simulink model "VSG_2M"  (R2022b)
settings: Solver=FixedStepAuto  StartTime=0.0  StopTime=2  FixedStep=1e-6  RelTol=1e-3
model workspace (MAT data in the model file):
  C = 0.0003
  D = 500
  GP = 0.6
  GQ = 20
  J = 2
  KQ = 0.06
  Kf = 80000
  Kv = 577
  L = 0.001
  Pref = 2000000
  Qref = 0
  Ts = 0.0001
  Ts_Power = 1e-06
  Ug = 400
  Vdc = 1000
  fsw = 20000
  t0 = 0.5
  tco = 1.3
  tf = 1.2
  wn = 314.159265359
undefined symbols (not defined in the file): DiscIntNeverNeededParam, Ion, Lithium
libraries: spsSeriesRLCBranchLib x8, spsFirstOrderFilterLib x7, spsMeanLib x5, slpidlib x5, spsabctodq0Lib x4, spsStairGeneratorLib x4, spsDiodeLib x4, spsPWMGeneratorDCDCLib x3, spsThreePhaseVIMeasurementLib x3, spsThreePhaseSeriesRLCBranchLib x3, spsPowerPositiveSequenceLib x2, spsBoostConverterLib x2
(part 2 of 2)

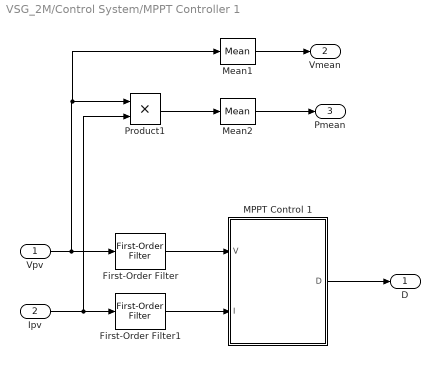
== system VSG_2M/Control System/MPPT Controller 1 ==
  Vpv : Inport
  Ipv : Inport  Port=2
  First-Order Filter : spsFirstOrderFilterLib/First-Order Filter  FilterType=Lowpass  Tc=1/Fc  Ts=Ts  Initialize=off  Vac_Init=[0, 0, 60]  Vdc_Init=0  PlotResponse=off  FreqRange="[0,  200,  1]"
  First-Order Filter1 : spsFirstOrderFilterLib/First-Order Filter  FilterType=Lowpass  Tc=1/Fc  Ts=Ts  Initialize=off  Vac_Init=[0, 0, 60]  Vdc_Init=0  PlotResponse=off  FreqRange="[0,  200,  1]"
  "MPPT Control 1 " : MATLAB Function  TreatAsAtomicUnit=on
  Mean1 : spsMeanLib/Mean  Freq=60  Vinit=650  Ts=Ts
  Mean2 : spsMeanLib/Mean  Freq=60  Vinit=1500e3  Ts=Ts
  Product1 : Product
  D : Outport  VectorParamsAs1DForOutWhenUnconnected=off
  Vmean : Outport  Port=2  VectorParamsAs1DForOutWhenUnconnected=off
  Pmean : Outport  Port=3  VectorParamsAs1DForOutWhenUnconnected=off
  wires:
  First-Order Filter1/1 -> "MPPT Control 1 "/2(I)
  First-Order Filter/1 -> "MPPT Control 1 "/1(V)
  Ipv/1 -> Product1/2, First-Order Filter1/1
  Vpv/1 -> Mean1/1, Product1/1, First-Order Filter/1
  "MPPT Control 1 "/1(D) -> D/1
  Product1/1 -> Mean2/1
  Mean1/1 -> Vmean/1
  Mean2/1 -> Pmean/1

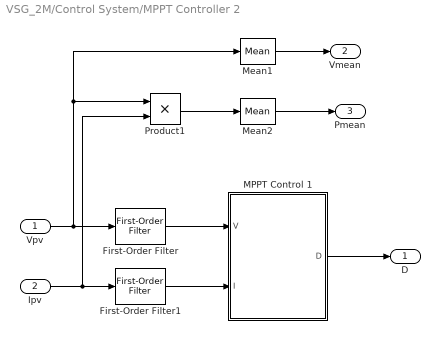
== system VSG_2M/Control System/MPPT Controller 2 ==
  Vpv : Inport
  Ipv : Inport  Port=2
  First-Order Filter : spsFirstOrderFilterLib/First-Order Filter  FilterType=Lowpass  Tc=1/Fc  Ts=Ts  Initialize=off  Vac_Init=[0, 0, 60]  Vdc_Init=0  PlotResponse=off  FreqRange="[0,  200,  1]"
  First-Order Filter1 : spsFirstOrderFilterLib/First-Order Filter  FilterType=Lowpass  Tc=1/Fc  Ts=Ts  Initialize=off  Vac_Init=[0, 0, 60]  Vdc_Init=0  PlotResponse=off  FreqRange="[0,  200,  1]"
  "MPPT Control 1 " : MATLAB Function  TreatAsAtomicUnit=on
  Mean1 : spsMeanLib/Mean  Freq=60  Vinit=420  Ts=Ts
  Mean2 : spsMeanLib/Mean  Freq=60  Vinit=500e3  Ts=Ts
  Product1 : Product
  D : Outport  VectorParamsAs1DForOutWhenUnconnected=off
  Vmean : Outport  Port=2  VectorParamsAs1DForOutWhenUnconnected=off
  Pmean : Outport  Port=3  VectorParamsAs1DForOutWhenUnconnected=off
  wires:
  "MPPT Control 1 "/1(D) -> D/1
  Ipv/1 -> Product1/2, First-Order Filter1/1
  First-Order Filter/1 -> "MPPT Control 1 "/1(V)
  First-Order Filter1/1 -> "MPPT Control 1 "/2(I)
  Mean1/1 -> Vmean/1
  Product1/1 -> Mean2/1
  Mean2/1 -> Pmean/1
  Vpv/1 -> Product1/1, Mean1/1, First-Order Filter/1

== system VSG_2M/光伏阵列/Subsystem1 ==

== system VSG_2M/光伏阵列/Subsystem2 ==

== matlab function VSG_2M/Control System/MPPT Controller 2/MPPT Control 1  ==
  settings: updateMethod=DISCRETE  sampleTime=Ts
  data: V input =V; I input; D output; Dmax parameter; Dmin parameter; deltaD parameter; Dinit parameter
function D  = PandO(V, I, Dmax, Dmin, deltaD, Dinit)

% MPPT controller based on the Perturb & Observe algorithm.

% D output = Duty cycle of the boost converter (value between 0 and 1)
% V input = PV array terminal voltage (V)
% I input = PV array current (A)
% D = 1 - Vinput/Voutput (increasing D decrease Vin)

persistent Vold Pold Dold;
%
if isempty(Vold)
    Vold=0;
    Pold=0;
    Dold=Dinit;
end
P= V*I;
dV= V - Vold;
dP= P - Pold;
%
% if dP ~= 0
    if dP < 0
        if dV < 0
            D = Dold - deltaD;
        else
            D = Dold + deltaD;
        end
    else
        if dV < 0
            D = Dold + deltaD;
        else
            D = Dold - deltaD;
        end    
    end
% else
%     D=Dold;
% end
%
if D >= Dmax || D<= Dmin
    D=Dold;
end
%
Dold=D;
Vold=V;
Pold=P;

== matlab function VSG_2M/Control System/MPPT Controller 1/MPPT Control 1  ==
  settings: updateMethod=DISCRETE  sampleTime=Ts
  data: V input =V; I input; D output; Dmax parameter; Dmin parameter; deltaD parameter; Dinit parameter
function D  = PandO(V, I, Dmax, Dmin, deltaD, Dinit)

% MPPT controller based on the Perturb & Observe algorithm.

% D output = Duty cycle of the boost converter (value between 0 and 1)
% V input = PV array terminal voltage (V)
% I input = PV array current (A)
% D = 1 - Vinput/Voutput (increasing D decrease Vin)

persistent Vold Pold Dold;
%
if isempty(Vold)
    Vold=0;
    Pold=0;
    Dold=Dinit;
end
P= V*I;
dV= V - Vold;
dP= P - Pold;
%
% if dP ~= 0
    if dP < 0
        if dV < 0
            D = Dold - deltaD;
        else
            D = Dold + deltaD;
        end
    else
        if dV < 0
            D = Dold + deltaD;
        else
            D = Dold - deltaD;
        end    
    end
% else
%     D=Dold;
% end
%
if D >= Dmax || D<= Dmin
    D=Dold;
end
%
Dold=D;
Vold=V;
Pold=P;
